simulink model "Pointmass_eom_v1_0_R2018B"  (R2018b)
settings: Solver=ode4  StartTime=0.0  StopTime=simInit.TSIM  FixedStep=simInit.dt  MaxStep=simInit.dt  RelTol=1e-3
InitFcn:
  | close all
undefined symbols (not defined in the file or in its folder): base_windspeed, constr, DE2019, DiscIntNeverNeededParam, ENVMT, Lbooth, loiterStates, params, simInit, T
libraries: simulink x26, simulink_extras x2, aerolibconvert2 x1, aerolibwind2 x1
(part 4 of 4)

== matlab function Pointmass_eom_v1_0_R2018B/AirborneSystem/FlightControlSystem/PathFollowingController/FlightOnFlatEarth (Retraction&Loitering)/GuidanceFlatEarth/Retraction_Nav/calculateTransitionTrigger1 ==
  data: d_gt output; d output; chi_k_cmd output; flag_pos_y_W output; switch_WP_x_W output; gamma_k_cmd output; pos_init_retraction_O input; pos_G_O_m input; transition_flag output; ENVMT parameter; v_k_tot input; constr parameter; params parameter; retraction_side input; vk_xy input; transition_flag_old input
% Copyright 2020 Delft University of Technology
%
% Licensed under the Apache License, Version 2.0 (the "License");
% you may not use this file except in compliance with the License.
% You may obtain a copy of the License at
%
%      http://www.apache.org/licenses/LICENSE-2.0
%
% Unless required by applicable law or agreed to in writing, software
% distributed under the License is distributed on an "AS IS" BASIS,
% WITHOUT WARRANTIES OR CONDITIONS OF ANY KIND, either express or implied.
% See the License for the specific language governing permissions and
% limitations under the License.

function [d_gt, d, chi_k_cmd,flag_pos_y_W,switch_WP_x_W, gamma_k_cmd, transition_flag] = ...
    slope_navigator(pos_init_retraction_O, pos_G_O_m, ENVMT, v_k_tot, constr, params, ...
    retraction_side, vk_xy, transition_flag_old)
%slope_navigator - Navigation on slope during retraction
%
% Inputs:
%    pos_init_retraction_O  - Aircraft position at start of retraction in
%                             inertial reference frame
%    pos_G_O_m              - Aircraft position in inertial reference frame
%    ENVMT                  - Environment characteristics
%    v_k_tot                - Magnitude of kinetic velocity
%    constr                 - Constraint, minimum altitude
%    params                 - Controller parameters and Fig8 shape
%    retraction_side        - Longtitude rate of change, used for positive,
%                             negative check
%    vk_xy                  - Horizontal kinetic velocity magnitude in wind
%                             reference frame
%    transition_flag_old    - Old transition from retraction to traction flag
%
% Outputs:
%    d_gt            - Distance to ground track
%    d               - Distance to slope
%    chi_k_cmd       - Desired Course angle
%    flag_pos_y_W    - Flag to determine on which side it needs to go into
%                      traction
%    switch_WP_x_W   - X coordinate of the retraction target to transition
%    gamma_k_cmd     - Desired path angle
%    transition_flag - Transition from retraction to traction flag
%
%
% Author: Sebastian Rapp, Ph.D., Revised by: Dylan Eijkelhof, M.Sc.
% Delft University of Technology
% email address: s.rapp@tudelft.nl
% email address: d.eijkelhof@tudelft.nl
% December 2019; Last revision: 07-October-2020

%-------------	BEGIN CODE	--------------

pos_init_retraction_W = transformFromOtoW(ENVMT.windDirection_rad, pos_init_retraction_O);

if retraction_side > 0 
    flag_pos_y_W = 1;
else
    flag_pos_y_W = 0;
end

%% outer point lemniscate
Lbooth.b = params.b_booth;
Lbooth.a = params.b_booth*params.a_booth;
Lbooth.phi0 = params.transition_phi*pi/180;
[Lem] = updateBoothLemniscate(params.l_tether_min,Lbooth);
if flag_pos_y_W
    s = pi/2;
else
    s = 3/2*pi; 
end
long_P = Lem.b * sin(s) ./( 1+(Lem.a/Lem.b*cos(s)).^2 );
lat_P =   Lem.a * sin(s).*cos(s) ./ ( 1+(Lem.a/Lem.b*cos(s)).^2 );
p_P = [ cos(long_P).*cos(lat_P);sin(long_P).*cos(lat_P);sin(lat_P)]*params.l_tether_min;
M_WP = [cos(Lbooth.phi0),0, -sin(Lbooth.phi0);0, 1, 0;  sin(Lbooth.phi0),0, cos(Lbooth.phi0)];  
p_W = M_WP * p_P; 
%%

target_W = p_W;% params.target_retraction_W;
r = params.r_retraction;
pos_W = transformFromOtoW(ENVMT.windDirection_rad, pos_G_O_m);

dx = pos_init_retraction_W(1) - target_W(1);
dy = pos_init_retraction_W(2) - target_W(2);
theta = atan( dy / dx );
alpha = pi/4+theta/2;
x_c_W = target_W(1) + r;
y_c_W = target_W(2) - 1/tan(alpha)*r;%cos(theta)*r;

switch_WP_x_W = p_W(1);%x_c_W - sin(theta)*r;
switch_WP_y_W = p_W(2);%y_c_W + cos(theta)*r;


switch_WP_W = [switch_WP_x_W;switch_WP_y_W;0];

if pos_W(1) <= p_W(1)+10 || transition_flag_old %pos_W(1) <= switch_WP_x_W || transition_flag_old 
    transition_flag = 1;
    pos_C = [pos_W(1); pos_W(2); 0] - [x_c_W;y_c_W;0];
    p_proj_C = pos_C/norm(pos_C)*r;
    d_gt = norm( pos_C - p_proj_C );
    s  = atan2( p_proj_C(2),p_proj_C(1) );
        
    t_W = [-sin(s); cos(s);0];
    t_O = transformFromWtoO(ENVMT.windDirection_rad, t_W);
    chi_star = atan2( t_O(2), t_O(1) );
    delta_chi = -asin( max( min( params.kp_delta_course*d_gt /vk_xy, 1), -1) ) * sign(norm(pos_C)-r);

    chi_k_cmd = chi_star + delta_chi;
    
    % wrap around +/- pi
    if chi_k_cmd > pi
        du = mod(chi_k_cmd,pi);
        chi_k_cmd = -pi+du;
    elseif chi_k_cmd < -pi
        du = mod(chi_k_cmd,-pi);
        chi_k_cmd = pi+du;
    else
        %
    end
else
    transition_flag = 0;
    groundtrack_bearing_W = target_W - pos_init_retraction_W;
    groundtrack_bearing_O = transformFromWtoO(ENVMT.windDirection_rad, groundtrack_bearing_W);
    chi_k_cmd = atan2( groundtrack_bearing_O(2), groundtrack_bearing_O(1) );
    
    % Desired ground track
    groundtrack_bearing_W(3) = 0;
    
    % relative position
    pos_rel_gt_W = pos_W - pos_init_retraction_W;
    pos_rel_gt_W(3) = 0;
    
    % projection onto groundtrack
    p_proj_W = pos_rel_gt_W'*groundtrack_bearing_W / norm( groundtrack_bearing_W )^2 * groundtrack_bearing_W;
    % distance 2 ground track
    d_gt = norm( pos_rel_gt_W - p_proj_W );
    z = cross( groundtrack_bearing_W,pos_rel_gt_W );
    
    delta_chi = sign(z(3)) * asin( max( min( params.kp_delta_course*d_gt / vk_xy, 1),-1) );
    
    chi_k_cmd = chi_k_cmd + delta_chi;
end

%% arc length of transition circle until transition point 

% min tether length before the turn
z_transition = max( sqrt( params.l_tether_min^2 - switch_WP_x_W^2 - switch_WP_y_W^2 ), constr.min_altitude_pc); % min. attitude has higher priority then min. tether length
dh = pos_init_retraction_W(3) - z_transition;
ds = sqrt( ( switch_WP_x_W - pos_init_retraction_W(1))^2 +  ( switch_WP_y_W - pos_init_retraction_W(2))^2 ); 
gamma_k_star =  -atan( dh/ds );

gs_direction_W = [switch_WP_W(1) - pos_init_retraction_W(1);switch_WP_W(2) - pos_init_retraction_W(2);-dh];

% Current relative position vector
p_rel_W = pos_W - pos_init_retraction_W;

% projection onto retraction slope
p_proj_W = p_rel_W'*gs_direction_W / norm( gs_direction_W )^2 * gs_direction_W;

% distance to slope
d = norm( p_rel_W - p_proj_W );

if transition_flag
    % check if above or below glide slope
    if pos_W(3) > z_transition
        sign_deltaGamma = 1;
    else
        sign_deltaGamma = -1;
    end
    d = abs( pos_W(3) - z_transition );
    gamma_k_star = 0;
else 
    % check if above or below glide slope
    z = cross( gs_direction_W,p_rel_W );
    sign_deltaGamma = sign(z(2));
end

gamma_k_cmd = gamma_k_star - asin( max( min(params.kp_delta_gamma*d*sign_deltaGamma/(v_k_tot+1e-3), pi/6), -pi/6) );

%-------------	 END CODE	--------------
end

== matlab function Pointmass_eom_v1_0_R2018B/RequirementModelsAndLogging/Power_convergence/MATLAB Function ==
  data: flag output; m_new output; p_sum output; cnt output; flag input; m_old input; p_sum input; cnt input; u input; flightMode input; e_new output; e_old input; cnt_max_mat input; cnt_max_mat output; cycles_cnt input; cycles_cnt output
% Copyright 2020 Delft University of Technology
%
% Licensed under the Apache License, Version 2.0 (the "License");
% you may not use this file except in compliance with the License.
% You may obtain a copy of the License at
%
%      http://www.apache.org/licenses/LICENSE-2.0
%
% Unless required by applicable law or agreed to in writing, software
% distributed under the License is distributed on an "AS IS" BASIS,
% WITHOUT WARRANTIES OR CONDITIONS OF ANY KIND, either express or implied.
% See the License for the specific language governing permissions and
% limitations under the License.

function [flag, m_new, p_sum, cnt, e_new, cnt_max_mat,cycles_cnt] = fcn(flag,m_old, p_sum, cnt,u, flightMode, e_old,cnt_max_mat,cycles_cnt)
%y = [u;old(1:end-1)];
% if cnt > nmax
%     new_mean = mean(y);
%     cnt = 0;
% end
p_sum = p_sum + u;
cnt = cnt + 1;

if flightMode == 5 && flag
    cnt_max_mat = cnt; 
    m_new = p_sum/cnt;
    cnt  = 0;
    cycles_cnt = cycles_cnt + 1;
    p_sum = 0;
    flag = 0;
    e_new = abs( m_new - m_old );
elseif flightMode == 6 
    flag = 1;
    m_new = m_old;
    e_new = e_old;
else
    flag = 0;
    m_new = m_old;
    e_new = e_old;
end

% m_new = m_old + (u-old(nmax))/nmax;

== matlab function Pointmass_eom_v1_0_R2018B/AirborneSystem/FlightControlSystem/PathFollowingController/FlightOnSphere (Traction)/FlightPathLoopTraction/EstimatePlantResponse/MATLAB Function ==
  data: F_t input; dphi input; mu_k input; chi_dot_real output; gamma_dot_real output; DE2019 parameter; chi_k input; gamma_k input; pos_O input; v_k_B input; airdata input; ENVMT parameter
% Copyright 2020 Delft University of Technology
%
% Licensed under the Apache License, Version 2.0 (the "License");
% you may not use this file except in compliance with the License.
% You may obtain a copy of the License at
%
%      http://www.apache.org/licenses/LICENSE-2.0
%
% Unless required by applicable law or agreed to in writing, software
% distributed under the License is distributed on an "AS IS" BASIS,
% WITHOUT WARRANTIES OR CONDITIONS OF ANY KIND, either express or implied.
% See the License for the specific language governing permissions and
% limitations under the License.

function [chi_dot_real, gamma_dot_real] = est_pathangles(F_t, dphi, mu_k,DE2019,chi_k,gamma_k, pos_O, v_k_B, airdata,ENVMT)
%est_pathangles - Estimate plant response
%
% Inputs:
%    F_t     - Tether set point
%    dphi    - Set to 0, not used currently
%    mu_k    - Roll angle
%    DE2019  - Aircraft characteristics
%    chi_k   - Course angle
%    gamma_k - Path angle
%    pos_O   - Aircraft position in inertial reference frame
%    v_k_B   - Kinetic velocity in body reference frame
%    airdata - Airspeed, aoa, sideslip
%    ENVMT   - Enivronment characteristics
%
% Outputs:
%    chi_dot_real    - Course angle rate of change
%    gamma_dot_real  - Path angle rate of change
%
%
% Author: Sebastian Rapp, Ph.D., Revised by: Dylan Eijkelhof, M.Sc.
% Delft University of Technology
% email address: s.rapp@tudelft.nl
% email address: d.eijkelhof@tudelft.nl
% December 2019; Last revision: 06-October-2020

%-------------	BEGIN CODE	--------------

Va = airdata(1); 
alpha = airdata(2); 
vk = norm(v_k_B); 
CL = DE2019.CL0 + DE2019.CL_alpha*alpha; 

Lrq = 0.5 * Va^2 * 1.225 * DE2019.S_wing * CL; 

c_chi_k = cos(chi_k); 
c_gamma_k = cos(gamma_k); 
s_chi_k = sin(chi_k); 
s_gamma_k = sin(gamma_k); 


M_KO = [ c_chi_k*c_gamma_k, s_chi_k*c_gamma_k, -s_gamma_k; 
    -s_chi_k, c_chi_k, 0; 
    c_chi_k*s_gamma_k, s_chi_k*s_gamma_k, c_gamma_k];

F_g_t_K = M_KO * ( [0;0;DE2019.mass*ENVMT.g] -F_t*pos_O/norm(pos_O) );

f_bar_z_K = -Lrq/sqrt(1+(tan(mu_k-dphi))^2); 

f_bar_y_K = -f_bar_z_K * tan( mu_k - dphi );

chi_dot_real = 1/cos(gamma_k)/vk/DE2019.mass  * ( f_bar_y_K + F_g_t_K(2) );
gamma_dot_real = -1/vk/DE2019.mass * ( f_bar_z_K + F_g_t_K(3) );

%-------------	 END CODE	--------------
end

== matlab function Pointmass_eom_v1_0_R2018B/AirborneSystem/FlightControlSystem/PathFollowingController/FlightOnSphere (Traction)/FlightPathLoopTraction/MATLAB Function ==
  data: L_rq output; airdata input; DE2019 parameter; constr parameter
% Copyright 2020 Delft University of Technology
%
% Licensed under the Apache License, Version 2.0 (the "License");
% you may not use this file except in compliance with the License.
% You may obtain a copy of the License at
%
%      http://www.apache.org/licenses/LICENSE-2.0
%
% Unless required by applicable law or agreed to in writing, software
% distributed under the License is distributed on an "AS IS" BASIS,
% WITHOUT WARRANTIES OR CONDITIONS OF ANY KIND, either express or implied.
% See the License for the specific language governing permissions and
% limitations under the License.

function L_rq = fcn(airdata, DE2019,constr)
%fcn - Calculate required lift force
%
% Inputs:
%    airdata     - Airspeed, aoa, sideslip angle
%    DE2019     - Aircraft characteristics
%    constr     - Constraint, maximum lift
%
% Outputs:
%    L_rq    - Required lift
%
% Author: Sebastian Rapp, Ph.D., Revised by: Dylan Eijkelhof, M.Sc.
% Delft University of Technology
% email address: s.rapp@tudelft.nl
% email address: d.eijkelhof@tudelft.nl
% December 2019; Last revision: 06-October-2020

%-------------	BEGIN CODE	--------------
L_rq =  min( 0.5*DE2019.rho_air*DE2019.S_wing*airdata(1)^2 * (DE2019.CL0+DE2019.CL_alpha*airdata(2) ),constr.F_T_max); % max. negative lift
%-------------	 END CODE	--------------
end

== matlab function Pointmass_eom_v1_0_R2018B/AirborneSystem/FlightControlSystem/PathFollowingController/FlightOnSphere (Traction)/FlightPathLoopTraction/inversionPathDynamics ==
  data: Ft_set input; nu_chi_k input; mu_a output; nu_gamma_k input; F_a_B_est input; DE2019 parameter; pos_O input; chi_k input; gamma_k input; v_k_B input; airdata input; constr parameter; mu_k_c output; alpha_rq output; dphi output; L_rq output; L_rq_old input; mu_a_old input; ENVMT parameter
% Copyright 2020 Delft University of Technology
%
% Licensed under the Apache License, Version 2.0 (the "License");
% you may not use this file except in compliance with the License.
% You may obtain a copy of the License at
%
%      http://www.apache.org/licenses/LICENSE-2.0
%
% Unless required by applicable law or agreed to in writing, software
% distributed under the License is distributed on an "AS IS" BASIS,
% WITHOUT WARRANTIES OR CONDITIONS OF ANY KIND, either express or implied.
% See the License for the specific language governing permissions and
% limitations under the License.

function [mu_a,mu_k_c,alpha_rq,dphi,L_rq] = InversePathDynamics(  Ft_set,nu_chi_k, nu_gamma_k, F_a_B_est,DE2019,pos_O,...
     chi_k, gamma_k, v_k_B, airdata,constr, L_rq_old, mu_a_old,ENVMT)
%InversePathDynamics - Calculated desired roll and pitch angles 
%
% Inputs:
%    Ft_set     - Tether force set point
%    nu_chi_k   - Course angle error
%    nu_gamma_k - Path angle error
%    F_a_B_est  - Aerodynamic forces in body reference frame
%    DE2019     - Aircraft characteristics
%    pos_O      - Aircraft position in inertial reference frame
%    chi_k      - Course angle
%    gamma_k    - Path angle
%    v_k_B      - Kinetic velocity
%    airdata    - Airspeed, aoa and sideslip angle
%    constr     - Dynamic constraints
%    L_rq_old   - Old required lift
%    mu_a_old   - Old roll angle
%    ENVMT      - Environment characteristics
%
% Outputs:
%    mu_a     - Desired aerodynamic roll angle
%    mu_k_c   - Kinetic roll angle
%    alpha_rq - Desired pitch angle
%    dphi     - Currently set to 0, not used anymore
%    L_rq     - Required lift
%
% Author: Sebastian Rapp, Ph.D., Revised by: Dylan Eijkelhof, M.Sc.
% Delft University of Technology
% email address: s.rapp@tudelft.nl
% email address: d.eijkelhof@tudelft.nl
% December 2019; Last revision: 06-October-2020

%-------------	BEGIN CODE	--------------
%% Initialise parameters for codegen
mu_a = 0;
mu_k_c = 0;
alpha_rq = 0;
dphi = 0;
v_k = 0;
L_rq = 0;
fbar_z_K = 0;
fbar_z_K_is = 0;

%%
f_t = Ft_set; 
mu_k_max = constr.mu_k_max;

beta_a = airdata(3); 

alpha_k = asin( v_k_B(3)/norm(v_k_B) ); 
beta_k = atan2( v_k_B(2), v_k_B(1) ); 

v_k = norm(v_k_B); 

c_chi_k = cos(chi_k); 
c_gamma_k = cos(gamma_k); 
s_chi_k = sin(chi_k); 
s_gamma_k = sin(gamma_k); 


M_KO = [ c_chi_k*c_gamma_k, s_chi_k*c_gamma_k, -s_gamma_k; 
    -s_chi_k, c_chi_k, 0; 
    c_chi_k*s_gamma_k, s_chi_k*s_gamma_k, c_gamma_k];

f_a_x_B = F_a_B_est(1); 
f_a_y_B = F_a_B_est(2); 
f_a_z_B = F_a_B_est(3); 


f_a_y_Kbar = -cos(alpha_k)*sin(beta_k)*f_a_x_B + cos(beta_k)*f_a_y_B - sin(alpha_k)*sin(beta_k)*f_a_z_B; 
f_a_z_Kbar = -sin(alpha_k)*f_a_x_B + cos(alpha_k)*f_a_z_B; 

f_t_K = -M_KO * pos_O/norm(pos_O)*f_t; 

fbar_y_K = DE2019.mass*nu_chi_k*cos(gamma_k)*v_k - f_t_K(2); 
fbar_z_K = -DE2019.mass*nu_gamma_k*v_k - cos(gamma_k)*DE2019.mass*ENVMT.g - f_t_K(3);

dphi = 0 * atan( f_a_y_Kbar / f_a_z_Kbar ); % this might be important at high wind speeds

mu_k_c = atan2( fbar_y_K, -fbar_z_K ) + dphi; 
fbar_y_K =  -fbar_z_K * tan( mu_k_c - dphi );

L_rq = min( sqrt( fbar_y_K^2 + fbar_z_K^2 )); % constraint by max. tether force e.g. structural limit

% limit mu_k: We do this for now directly: if we assume that the kite is in
% the tangential plane this corresponds well to the limits for phi_tau

mu_k_c = max( min( mu_k_c, mu_k_max), -mu_k_max); 

mu_a = mu_k_c;

% hold old bank angle if required lift is very small, avoid agressive
% banking for small absolute values of L i.e. for small values inaccuracies
% like numerical inaccuracies have a large impact on the mu_a_c.
if abs(L_rq) <= 10
    mu_a = mu_a_old;
end

% for large bank angle changes only adapt the lift if close to the current
% lift. The longitudional dynamic is faster, hence if we command large bank
% angles this would result in a large lift which would first create a large
% curvature in the longi plane before the actual curvature in the lateral
% plan is achieved.
if abs( mu_a - mu_a_old ) > constr.max_delta_mu
    L_rq = L_rq_old;
end

CL_rq = 2*L_rq / ( DE2019.rho_air*DE2019.S_wing*airdata(1)^2 );
alpha_rq = (CL_rq - DE2019.CL0)/DE2019.CL_alpha; 

%-------------	 END CODE	--------------
end

== matlab function Pointmass_eom_v1_0_R2018B/AirborneSystem/FlightControlSystem/PathFollowingController/FlightOnSphere (Traction)/Navigator/LissajousFigure8Following ==
  data: chi_k_ideal output; gamma_k_ideal output; chi_dot output; gamma_dot output; delta_ct output; pathAngles input; pos_W input; v_w_vec input; v_O_vec input; ENVMT parameter; long input; lat input; Lbooth parameter; params parameter; gamma_tau_dot input; gamma_tau_cmd input; PHI_BOOTH input; sol output; sol_old input
% Copyright 2020 Delft University of Technology
%
% Licensed under the Apache License, Version 2.0 (the "License");
% you may not use this file except in compliance with the License.
% You may obtain a copy of the License at
%
%      http://www.apache.org/licenses/LICENSE-2.0
%
% Unless required by applicable law or agreed to in writing, software
% distributed under the License is distributed on an "AS IS" BASIS,
% WITHOUT WARRANTIES OR CONDITIONS OF ANY KIND, either express or implied.
% See the License for the specific language governing permissions and
% limitations under the License.

function [chi_k_ideal, gamma_k_ideal, chi_dot, ...
    gamma_dot, delta_ct, sol] = fig8_navigator(pathAngles, ...
    pos_W,v_w_vec, v_O_vec, ENVMT, long, lat,Lbooth,params,gamma_tau_dot, ...
    gamma_tau_cmd,PHI_BOOTH, sol_old)
%fig8_navigator - Unlinke the other modules this module directly calculates
%                 the desired course and path angle rate
%
% Inputs:
%    pathAngles     - Course and path angles
%    pos_W          - Aircraft position in wind reference frame
%    v_w_vec        - Wind speed in wind reference frame
%    v_O_vec        - Kinetic velocity in inertial reference frame
%    ENVMT          - Environment characteristics
%    long           - Logtitude (ground station in sphere centre)
%    lat            - Latitude (ground station in sphere centre)
%    Lbooth         - Structure initialisation, parameters not used
%    params         - Controller parameters and Fig8 shape
%    gamma_tau_dot  - Input 0!
%    gamma_tau_cmd  - Input 0!
%    PHI_BOOTH      - Elevation angle
%    sol_old        - Old point on fig8 (0->2pi)
%
% Outputs:
%    chi_k_ideal     - Desired kinetic course angle
%    gamma_k_ideal   - Desired kinetic path angle
%    chi_dot         - Course angle rate of change
%    gamma_dot       - Path angle rate of change
%    delta_ct        - Cross-track error
%    sol             - Point on fig8 (0->2pi)
%
% Author: Sebastian Rapp, Ph.D., Revised by: Dylan Eijkelhof, M.Sc.
% Delft University of Technology
% email address: s.rapp@tudelft.nl
% email address: d.eijkelhof@tudelft.nl
% December 2019; Last revision: 06-October-2020

%-------------	BEGIN CODE	--------------

windDirection_rad = ENVMT.windDirection_rad;

b_booth = params.b_booth;
a_booth = params.a_booth;


% total kinematic velocity
Vtot = sqrt( v_O_vec'*v_O_vec );

% transform position from NEDframe (O) into Windframe (W)
phi_p_mean = PHI_BOOTH;  
M_WP = [cos(phi_p_mean),0, -sin(phi_p_mean);0, 1, 0; sin(phi_p_mean),0, cos(phi_p_mean)];
pos_P = M_WP' * pos_W; 

distanceOrigin = norm(pos_P);

% Booth Lemniscate
Lbooth.a = a_booth*b_booth; % height
Lbooth.b = b_booth; % length
Lbooth.phi0 = PHI_BOOTH; %phi0_booth*pi/180;

[Lem] = updateBoothLemniscate(distanceOrigin,Lbooth);
direction = -1;
[ sol,p_C_P] = getTargetOnBoothNewton2(Lem, pos_P, sol_old, distanceOrigin, direction);
[t_P,DtDs_P,~,~,~] = getBoothInfos2(sol,Lem, direction);
t = M_WP * t_P; 
DtDs = M_WP * DtDs_P; 
p_C_W = M_WP * p_C_P; 

% ---- I Think everything below is curve independent -----

% Step 2: Calculate distance to closest point
delta = acos( min( max( pos_W'/norm(pos_W) * p_C_W/norm(p_C_W), -1),1 ) );
delta_ct = delta * distanceOrigin;

% Step 3: Calculate the perpendicular course
[ ~, delta_vec, bearing_sign ] = calcCourse2ClosestPoint( p_C_W, pos_W );
delta_ct_signed = bearing_sign*delta;

% Step 3.5: Parallel transport of vectors at the path point to the kite
% position
t_rot = doRodriguesRotation(pos_W, p_C_W, t);
t_rot_T = transformFromWtoTau(long, lat, t_rot);
chi_parallel = atan2( t_rot_T(2), t_rot_T(1) );

chi = atan2( v_O_vec(2), v_O_vec(1) ); 
gamma = -asin( v_O_vec(3)/norm(v_O_vec) ); 
bearing_is_O = [cos(chi)*cos(gamma);
    sin(chi)*cos(gamma);
    -sin(gamma)];
bearing_is_tau = transformFromWtoTau( long, lat, transformFromOtoW(windDirection_rad, bearing_is_O));
chi_tau_is = atan2( bearing_is_tau(2), bearing_is_tau(1));
gamma_tau_is = -asin( bearing_is_tau(3) / norm( bearing_is_tau ) );

% Step 4: Calculate commanded course in tangential plane
% and determine the ideal bearing vector
V_k_tau = [cos(chi_tau_is)*cos(gamma_tau_is),sin(chi_tau_is)*cos(gamma_tau_is),0]*Vtot/distanceOrigin; 
delta0 = min(params.delta0_slope*norm(V_k_tau),0.1)+params.delta0_offset;%0.0025*max( min( norm(V_k_tau), 35),25) ;

[chi_tau, ~,~, Delta_chi_dot, ~] = calculateCommandedCourse2(t_rot,delta_vec, delta, delta0, chi_parallel, p_C_W, pos_W,v_w_vec, chi_tau_is);

% Step 5: Predict the required course rate due to the path curvature
[chi_tau_dot_predict] = predictChiDotRequ(long,lat,v_w_vec, pos_W,p_C_W, t, DtDs,chi_parallel );

gamma_tau = gamma_tau_cmd;

v_tau = [cos(chi_tau)*cos(gamma_tau); 
         sin(chi_tau)*cos(gamma_tau); 
        -sin(gamma_tau)]*Vtot;

v_w_vec_ideal = transformFromTautoW(long,lat, v_tau);
bearing_O = transformFromWtoO(windDirection_rad, v_w_vec_ideal); 
chi_k_ideal = atan2( bearing_O(2), bearing_O(1) ); 
gamma_k_ideal = -asin( bearing_O(3)/norm(bearing_O) ); 

% Step 6: Calculate the required course rate in the tangential plane 
nu_ref = chi_tau_dot_predict + Delta_chi_dot;

%%
chi = pathAngles(1); 
gamma = pathAngles(2);
chi_tau_dot_cmd = nu_ref ;

[chi_dot, gamma_dot] = getChiDotGammaDotOK(ENVMT.windDirection_rad,lat,long, v_w_vec,...
    chi_tau_dot_cmd, norm(pos_W),chi, gamma, v_w_vec_ideal, pos_W,gamma_tau,gamma_tau_dot);

%-------------	 END CODE	--------------
end

== matlab function Pointmass_eom_v1_0_R2018B/AirborneSystem/FlightControlSystem/PathFollowingController/FlightOnSphere (Traction)/Navigator/calcualteCourseErrorAndWrap1 ==
  data: chi_ref input; e_course output; chi input
% Copyright 2020 Delft University of Technology
%
% Licensed under the Apache License, Version 2.0 (the "License");
% you may not use this file except in compliance with the License.
% You may obtain a copy of the License at
%
%      http://www.apache.org/licenses/LICENSE-2.0
%
% Unless required by applicable law or agreed to in writing, software
% distributed under the License is distributed on an "AS IS" BASIS,
% WITHOUT WARRANTIES OR CONDITIONS OF ANY KIND, either express or implied.
% See the License for the specific language governing permissions and
% limitations under the License.

function e_course = course_error(chi_ref, chi)
%course_error - Calculate the error between commanded and actual course angle
%
% Inputs:
%    chi_ref  - Required chi
%    chi      - Actual chi
%
% Outputs:
%    e_course - Course (heading) error
%
% Example: 
%    
%
% Author: Sebastian Rapp, Ph.D., Revised by: Dylan Eijkelhof, M.Sc.
% Delft University of Technology
% email address: s.rapp@tudelft.nl
% email address: d.eijkelhof@tudelft.nl
% December 2019; Last revision: 06-October-2020

%-------------	BEGIN CODE	--------------
%#codegen
% The vectors are lying in the tangential plane attached to the current
% position on the small earth.
p_bearing_vec   = [cos(chi); sin(chi); 0];
p_bearing_vec   = p_bearing_vec/norm(p_bearing_vec); 

ref_bearing_vec = [cos(chi_ref); sin(chi_ref); 0];
ref_bearing_vec = ref_bearing_vec/norm(ref_bearing_vec); 

e_z = cross( ref_bearing_vec, p_bearing_vec ); 

dot_product = dot( ref_bearing_vec, p_bearing_vec ); 
if dot_product > 1 
	dot_product = 1; 
end
if dot_product < -1 
	dot_product = -1; 
end

e_course = - sign( e_z(3) ) * acos( max(min(dot_product,1),-1) );
%-------------	 END CODE	--------------
end

== matlab function Pointmass_eom_v1_0_R2018B/Environment/ShearWind/MATLAB Function ==
  data: v_w_u input; v_w_p_mat output
% Copyright 2020 Delft University of Technology
%
% Licensed under the Apache License, Version 2.0 (the "License");
% you may not use this file except in compliance with the License.
% You may obtain a copy of the License at
%
%      http://www.apache.org/licenses/LICENSE-2.0
%
% Unless required by applicable law or agreed to in writing, software
% distributed under the License is distributed on an "AS IS" BASIS,
% WITHOUT WARRANTIES OR CONDITIONS OF ANY KIND, either express or implied.
% See the License for the specific language governing permissions and
% limitations under the License.

function v_w_p_mat = fcn(v_w_u)

v_w_p_mat = zeros( 3, length( v_w_u) );
v_w_p_mat(1,:) = v_w_u';

== matlab function Pointmass_eom_v1_0_R2018B/AirborneSystem/FlightControlSystem/AirspeedController/Airspeed_Control/FeedforwardPart ==
  data: gamma input; T output; nu_V input; ENVMT parameter; Drag_force input; DE2019 parameter
% Copyright 2020 Delft University of Technology
%
% Licensed under the Apache License, Version 2.0 (the "License");
% you may not use this file except in compliance with the License.
% You may obtain a copy of the License at
%
%      http://www.apache.org/licenses/LICENSE-2.0
%
% Unless required by applicable law or agreed to in writing, software
% distributed under the License is distributed on an "AS IS" BASIS,
% WITHOUT WARRANTIES OR CONDITIONS OF ANY KIND, either express or implied.
% See the License for the specific language governing permissions and
% limitations under the License.

function T = feedforward_thrust(gamma, nu_V,  ENVMT, Drag_force, DE2019)
%feedforward_thrust - Thrust calculation for velocity initialisation
%
% Inputs:
%    gamma      - Path angle (glideslope)
%    nu_V       - Controlled velocity parameter
%    ENVMT      - Environmental characteristics
%    Drag_force	- Drag
%    DE2019     - Aircraft characteristics
%
% Outputs:
%    T          - Thrust force
%
% Example: 
%    T = feedforward_thrust(gamma, nu_V,  ENVMT, Drag_force, DE2019)
%
% Author: Sebastian Rapp, Ph.D., Revised by: Dylan Eijkelhof, M.Sc.
% Delft University of Technology
% email address: s.rapp@tudelft.nl
% email address: d.eijkelhof@tudelft.nl
% December 2019; Last revision: 06-October-2020

%-------------	BEGIN CODE	--------------

T = DE2019.mass * ( ENVMT.g * sin(gamma) + nu_V ) + Drag_force; % required thrust

% Based on the quotient of commmanded to max. available thrust
% F_T_max = ENVMT.rhos * DE2019.S_prop * DE2019.C_prop * DE2019.k_motor * (DE2019.k_motor - Va);
% delta_t = T/F_T_max; 

%-------------	 END CODE	--------------
end

== matlab function Pointmass_eom_v1_0_R2018B/AirborneSystem/FlightControlSystem/AirspeedController/Airspeed_Control/MATLAB Function ==
  data: F_a_B input; Drag output; AoA input
% Copyright 2020 Delft University of Technology
%
% Licensed under the Apache License, Version 2.0 (the "License");
% you may not use this file except in compliance with the License.
% You may obtain a copy of the License at
%
%      http://www.apache.org/licenses/LICENSE-2.0
%
% Unless required by applicable law or agreed to in writing, software
% distributed under the License is distributed on an "AS IS" BASIS,
% WITHOUT WARRANTIES OR CONDITIONS OF ANY KIND, either express or implied.
% See the License for the specific language governing permissions and
% limitations under the License.

function Drag = estimate_drag(F_a_B, AoA)

%estimate_drag - Transform drag from B to A reference frame
%
% Inputs:
%    F_a_B     - Aerodynamic forces in body reference frame
%    AoA       - Angle of Attack
%
% Outputs:
%    Drag    - Drag force
%
% Example: 
%    Drag = estimate_drag(F_a_B, AoA)
%
% Author: Sebastian Rapp, Ph.D., Revised by: Dylan Eijkelhof, M.Sc.
% Delft University of Technology
% email address: s.rapp@tudelft.nl
% email address: d.eijkelhof@tudelft.nl
% December 2019; Last revision: 06-October-2020

%-------------	BEGIN CODE	--------------

F_a_A = [cos(AoA), 0, sin(AoA);
    0, 1, 0; 
    -sin(AoA), 0, cos(AoA)] * F_a_B;

Drag = -F_a_A(1);

%-------------	 END CODE	--------------
end

== matlab function Pointmass_eom_v1_0_R2018B/AirborneSystem/FlightControlSystem/AirspeedController/Airspeed_Control/hedging ==
  data: Drag_force input; gamma input; nu_V output; T input; ENVMT parameter; DE2019 parameter
% Copyright 2020 Delft University of Technology
%
% Licensed under the Apache License, Version 2.0 (the "License");
% you may not use this file except in compliance with the License.
% You may obtain a copy of the License at
%
%      http://www.apache.org/licenses/LICENSE-2.0
%
% Unless required by applicable law or agreed to in writing, software
% distributed under the License is distributed on an "AS IS" BASIS,
% WITHOUT WARRANTIES OR CONDITIONS OF ANY KIND, either express or implied.
% See the License for the specific language governing permissions and
% limitations under the License.

function nu_V = hedgingV(Drag_force, gamma, T, ENVMT, DE2019)

%hedgingV
%
% Inputs:
%    Drag_force	- Drag
%    gamma      - Path angle (glideslope)
%    T          - Thrust force
%    ENVMT      - Environmental characteristics
%    DE2019     - Aircraft characteristics
%
% Outputs:
%    nu_V       - Controlled velocity parameter
%
% Example: 
%    nu_V = hedgingV(Drag_force, gamma, T, ENVMT, DE2019)
%
% Author: Sebastian Rapp, Ph.D., Revised by: Dylan Eijkelhof, M.Sc.
% Delft University of Technology
% email address: s.rapp@tudelft.nl
% email address: d.eijkelhof@tudelft.nl
% December 2019; Last revision: 06-October-2020

%-------------	BEGIN CODE	--------------

% Based on the quotient of commmanded to max. available thrust
% F_T_max = ENVMT.rhos * DE2019.S_prop * DE2019.C_prop * DE2019.k_motor * (DE2019.k_motor - Va);
% T = F_T_max * delta_t; 

nu_V = (T-Drag_force)/DE2019.mass - ENVMT.g * sin(gamma); 

%-------------	 END CODE	--------------
end

== stateflow chart Pointmass_eom_v1_0_R2018B/AirborneSystem/FlightControlSystem/AirspeedController/Chart ==
  state Throttle_Off
    entry: throttle_on = 0;
  state Throttle_On
    entry: throttle_on = 1;
  (default) -> Throttle_Off
  Throttle_Off -> Throttle_On : [Va<Va_min || manual_switch_on || init_throttle_flag]
  Throttle_On -> Throttle_Off : [Va>Va_min+10&&manual_switch_on==0&& init_throttle_flag ==0]
  data: Va input; Va_min input; init_throttle_flag input; throttle_on output; manual_switch_on input
